simulink library "fen"  (Simulink 8.1)
settings: Solver=ode1  StartTime=0.0  StopTime=Inf  FixedStep=0.001  RelTol=1e-3
PostLoadFcn:
  | , if any(exist('dsrtsu_mdlpostloadfcn', 'file') == [2, 3, 6]), try dsrtsu_mdlpostloadfcn('Execute', bdroot); catch fprintf('Error in PostLoadFcn (dsrtsu_mdlpostloadfcn) for model "%s":\n %s\n', bdroot, lasterr); end, end,
undefined symbols (not defined in the file or in its folder): ENUM_KEYSWITCH_ON, ENUM_SENSORSTATE_NORMAL, FALSE
settings Model: DSRTSU_INTERNAL_RTI_VER=450  DSRTSU_INTERNAL_RTI_TYPE=rti1401  RTICANMMDATA=struct('GeneralSetupData',struct('modelroot','D:\ELN150201_TAIWAN\trunk\AdasDragon\software\sw_development\arch\app\jud','generalsettings',struct('filesettings',struct('destfolder',struct('Name','RTICANMM_FILES','Check',1),'buildfolder',struct('Name','.','Check',1),'AbsDestfolder',struct('Name','D:\ELN150201_TAIWAN\trunk\AdasDragon\software\sw_development\arch\app\jud\RTICANMM_FILES'),'AbsBuildfolder',struct('Name','D:\ELN150201_TAIWAN\trunk\AdasDragon\software\sw_development\arch\app\jud'))),'options',struct('addpaths',1,'rmpaths',1,'addtrcexclusion',logical(1),'cannavigator',struct('checkmonitoring',0),'show_usrtrc',0,'use_usrtrc',0),'advanced',struct('options',[1 1 1 1 1 1 1 1 1 1 1 1 1 1 1 1 1 1 1 1 1 1 1 1 1 1 1 1 1 1 1 1 1 1 1 1 1 1 1 1 1 1 1 1 1 1 1 1 1 1 1 1 1 1 1 1 1 1 1 1 1 1 1 1 1 1 1 1 1 1 1 1 1 1 1 1 1 1 1 1 1 1 1 1 1 1 1 1 1 1 1 1 1 1 1 1 1 1 1 1]),'MPSetup',{{}},'modelname','fen','block','fen'))  DSRTSU_INTERNAL_RTIFPGA=40  Creator=AT015411  LastModifiedBy=AT015555

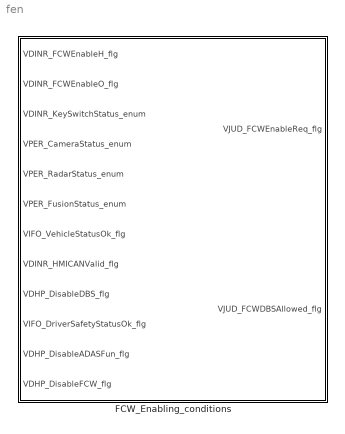
== system fen ==
  FCW_Enabling_conditions : Subsystem

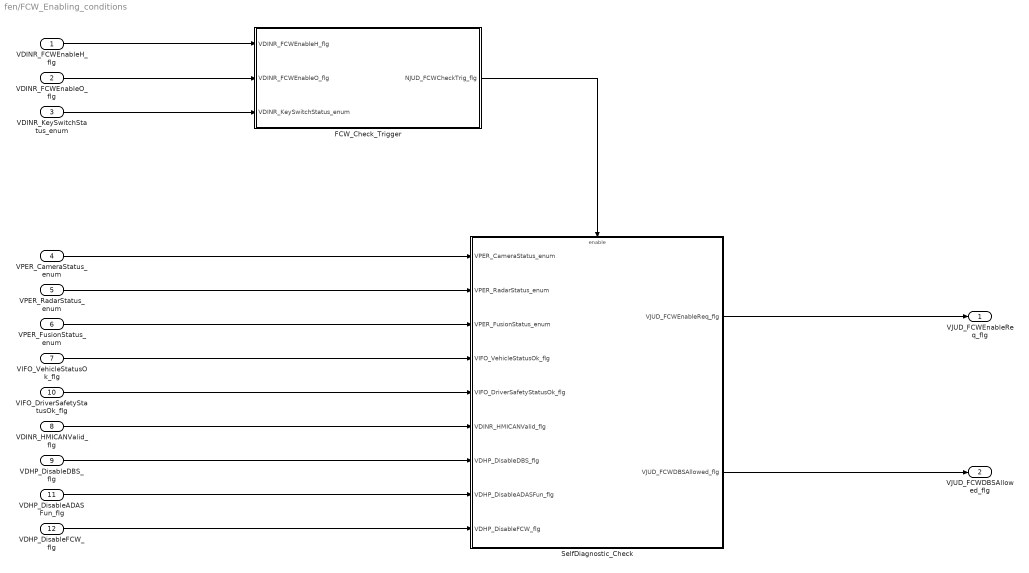
== system fen/FCW_Enabling_conditions ==
  VDINR_FCWEnableH_flg : Inport
  VDINR_FCWEnableO_flg : Inport  Port=2
  VDINR_KeySwitchStatus_enum : Inport  Port=3
  VPER_CameraStatus_enum : Inport  Port=4
  VPER_RadarStatus_enum : Inport  Port=5
  VPER_FusionStatus_enum : Inport  Port=6
  VIFO_VehicleStatusOk_flg : Inport  Port=7
  VDINR_HMICANValid_flg : Inport  Port=8
  VDHP_DisableDBS_flg : Inport  Port=9
  VIFO_DriverSafetyStatusOk_flg : Inport  Port=10
  VDHP_DisableADASFun_flg : Inport  Port=11
  VDHP_DisableFCW_flg : Inport  Port=12
  FCW_Check_Trigger : Subsystem
  SelfDiagnostic_Check : Subsystem
  VJUD_FCWEnableReq_flg : Outport
  VJUD_FCWDBSAllowed_flg : Outport  Port=2
  wires:
  VDHP_DisableADASFun_flg/1 -> SelfDiagnostic_Check/8(VDHP_DisableADASFun_flg)
  VDHP_DisableDBS_flg/1 -> SelfDiagnostic_Check/7(VDHP_DisableDBS_flg)
  VDHP_DisableFCW_flg/1 -> SelfDiagnostic_Check/9(VDHP_DisableFCW_flg)
  FCW_Check_Trigger/1(NJUD_FCWCheckTrig_flg) -> SelfDiagnostic_Check/Enable
  VDINR_KeySwitchStatus_enum/1 -> FCW_Check_Trigger/3(VDINR_KeySwitchStatus_enum)
  VDINR_FCWEnableO_flg/1 -> FCW_Check_Trigger/2(VDINR_FCWEnableO_flg)
  VDINR_FCWEnableH_flg/1 -> FCW_Check_Trigger/1(VDINR_FCWEnableH_flg)
  SelfDiagnostic_Check/2(VJUD_FCWDBSAllowed_flg) -> VJUD_FCWDBSAllowed_flg/1
  SelfDiagnostic_Check/1(VJUD_FCWEnableReq_flg) -> VJUD_FCWEnableReq_flg/1
  VIFO_DriverSafetyStatusOk_flg/1 -> SelfDiagnostic_Check/5(VIFO_DriverSafetyStatusOk_flg)
  VDINR_HMICANValid_flg/1 -> SelfDiagnostic_Check/6(VDINR_HMICANValid_flg)
  VIFO_VehicleStatusOk_flg/1 -> SelfDiagnostic_Check/4(VIFO_VehicleStatusOk_flg)
  VPER_FusionStatus_enum/1 -> SelfDiagnostic_Check/3(VPER_FusionStatus_enum)
  VPER_RadarStatus_enum/1 -> SelfDiagnostic_Check/2(VPER_RadarStatus_enum)
  VPER_CameraStatus_enum/1 -> SelfDiagnostic_Check/1(VPER_CameraStatus_enum)

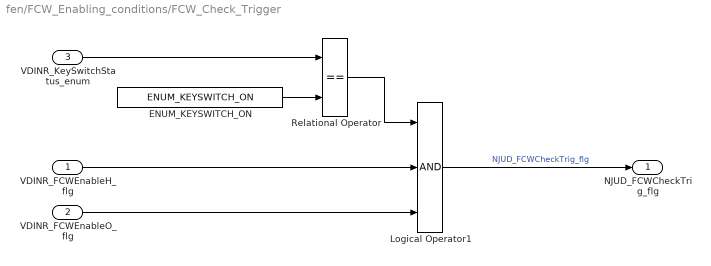
== system fen/FCW_Enabling_conditions/FCW_Check_Trigger ==
  VDINR_FCWEnableH_flg : Inport
  VDINR_FCWEnableO_flg : Inport  Port=2
  VDINR_KeySwitchStatus_enum : Inport  Port=3
  ENUM_KEYSWITCH_ON : Constant  Value=ENUM_KEYSWITCH_ON  OutDataTypeStr=uint8
  Logical Operator1 : Logic  Inputs=3  AllPortsSameDT=off  OutDataTypeStr=boolean
  Relational Operator : RelationalOperator  Operator===  OutDataTypeStr=boolean
  NJUD_FCWCheckTrig_flg : Outport
  wires:
  VDINR_FCWEnableO_flg/1 -> Logical Operator1/3
  VDINR_FCWEnableH_flg/1 -> Logical Operator1/2
  Logical Operator1/1 -> NJUD_FCWCheckTrig_flg/1  "NJUD_FCWCheckTrig_flg"
  Relational Operator/1 -> Logical Operator1/1
  VDINR_KeySwitchStatus_enum/1 -> Relational Operator/1
  ENUM_KEYSWITCH_ON/1 -> Relational Operator/2

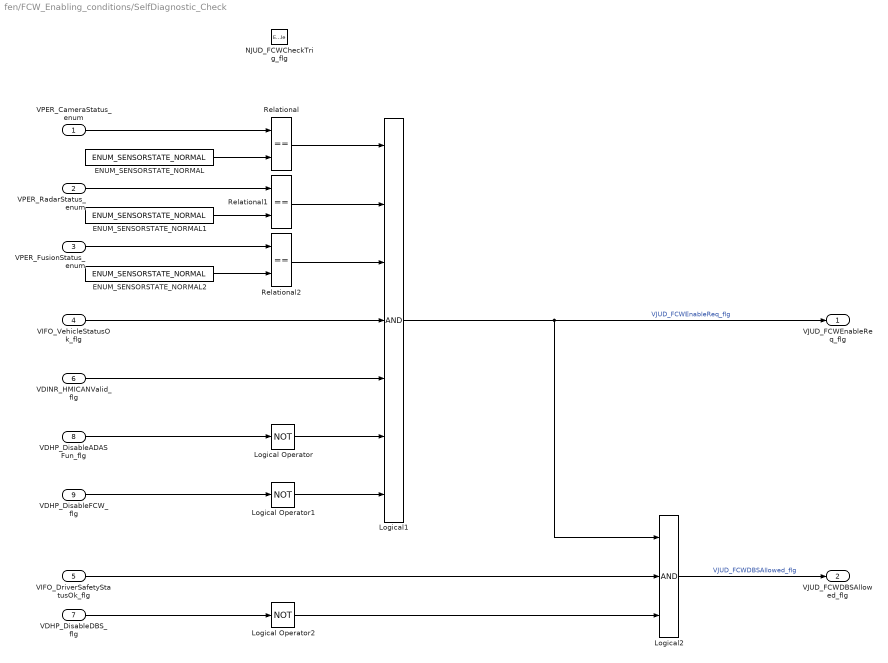
== system fen/FCW_Enabling_conditions/SelfDiagnostic_Check ==
  VPER_CameraStatus_enum : Inport
  VPER_RadarStatus_enum : Inport  Port=2
  VPER_FusionStatus_enum : Inport  Port=3
  VIFO_VehicleStatusOk_flg : Inport  Port=4
  VIFO_DriverSafetyStatusOk_flg : Inport  Port=5
  VDINR_HMICANValid_flg : Inport  Port=6
  VDHP_DisableDBS_flg : Inport  Port=7
  VDHP_DisableADASFun_flg : Inport  Port=8
  VDHP_DisableFCW_flg : Inport  Port=9
  NJUD_FCWCheckTrig_flg : EnablePort  StatesWhenEnabling=reset
      settings: AttributesFormatString=State =%<StatesWhenEnabling>
  ENUM_SENSORSTATE_NORMAL : Constant  Value=ENUM_SENSORSTATE_NORMAL  OutDataTypeStr=uint8
  ENUM_SENSORSTATE_NORMAL1 : Constant  Value=ENUM_SENSORSTATE_NORMAL  OutDataTypeStr=uint8
  ENUM_SENSORSTATE_NORMAL2 : Constant  Value=ENUM_SENSORSTATE_NORMAL  OutDataTypeStr=uint8
  Logical Operator : Logic  Operator=NOT  AllPortsSameDT=off  OutDataTypeStr=boolean
  Logical Operator1 : Logic  Operator=NOT  AllPortsSameDT=off  OutDataTypeStr=boolean
  Logical Operator2 : Logic  Operator=NOT  AllPortsSameDT=off  OutDataTypeStr=boolean
  Logical1 : Logic  Inputs=7  AllPortsSameDT=off  OutDataTypeStr=boolean
  Logical2 : Logic  Inputs=3  AllPortsSameDT=off  OutDataTypeStr=boolean
  Relational : RelationalOperator  Operator===  OutDataTypeStr=boolean
  Relational1 : RelationalOperator  Operator===  OutDataTypeStr=boolean
  Relational2 : RelationalOperator  Operator===  OutDataTypeStr=boolean
  VJUD_FCWEnableReq_flg : Outport  OutputWhenDisabled=reset  InitialOutput=FALSE
  VJUD_FCWDBSAllowed_flg : Outport  Port=2  OutputWhenDisabled=reset  InitialOutput=FALSE
  wires:
  Logical Operator2/1 -> Logical2/3
  Logical Operator1/1 -> Logical1/7
  Logical Operator/1 -> Logical1/6
  VDHP_DisableDBS_flg/1 -> Logical Operator2/1
  VDHP_DisableFCW_flg/1 -> Logical Operator1/1
  VDHP_DisableADASFun_flg/1 -> Logical Operator/1
  ENUM_SENSORSTATE_NORMAL2/1 -> Relational2/2
  VPER_FusionStatus_enum/1 -> Relational2/1
  Relational2/1 -> Logical1/3
  ENUM_SENSORSTATE_NORMAL1/1 -> Relational1/2
  VPER_RadarStatus_enum/1 -> Relational1/1
  Logical2/1 -> VJUD_FCWDBSAllowed_flg/1  "VJUD_FCWDBSAllowed_flg"
  VIFO_DriverSafetyStatusOk_flg/1 -> Logical2/2
  Logical1/1 -> Logical2/1, VJUD_FCWEnableReq_flg/1  "VJUD_FCWEnableReq_flg"
  VIFO_VehicleStatusOk_flg/1 -> Logical1/4
  Relational1/1 -> Logical1/2
  Relational/1 -> Logical1/1
  VDINR_HMICANValid_flg/1 -> Logical1/5
  ENUM_SENSORSTATE_NORMAL/1 -> Relational/2
  VPER_CameraStatus_enum/1 -> Relational/1
